simulink model "testRef"  (R2025a)
settings: Solver=ode23t  StartTime=0.0  StopTime=10.0  RelTol=1e-3
settings Model: Creator=grouleau  LastModifiedBy=grouleau
settings ModelReferenceCC: UseModelRefSolver=on

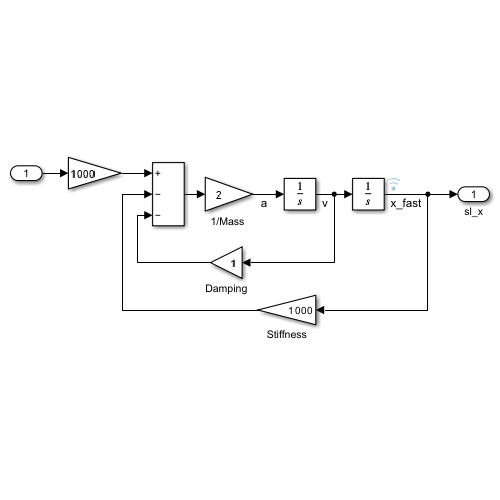
[thumbnail: Simulink's stored preview of the top-level diagram]
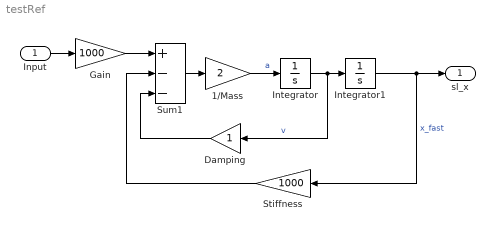
== system testRef ==
  Input : Inport
  "1/Mass " : Gain  Gain=2  SaturateOnIntegerOverflow=on  OutDataTypeStr=Inherit: Same as input  ParamDataTypeStr=Inherit: Same as input
  Damping : Gain
  Gain : Gain  Gain=1000
  Integrator : Integrator
  Integrator1 : Integrator
  Stiffness : Gain  Gain=1000  SaturateOnIntegerOverflow=on  OutDataTypeStr=Inherit: Same as input  ParamDataTypeStr=Inherit: Same as input
  Sum1 : Sum  Inputs=+--  InputSameDT=on  SaturateOnIntegerOverflow=on  OutDataTypeStr=Inherit: Same as first input
  sl_x : Outport
  wires:
  Stiffness/1 -> Sum1/2
  Integrator/1 -> Damping/1, Integrator1/1  "v"
  Sum1/1 -> "1/Mass "/1
  "1/Mass "/1 -> Integrator/1  "a"
  Damping/1 -> Sum1/3
  Integrator1/1 -> Stiffness/1, sl_x/1  "x_fast"
  Input/1 -> Gain/1
  Gain/1 -> Sum1/1
